simulink model "shunthybrid"  (Simulink 7.3)
settings: Solver=ode45  StartTime=0.0  StopTime=1.5  RelTol=1e-3
InitFcn:
  | Ts=50e-6;
StartFcn:
  | clear all
  | clc
  | Ts=2e-6
libraries: powerlib x35, powerlib_extras x7
settings Model: Creator=Anil  LastModifiedBy=SANTOSH

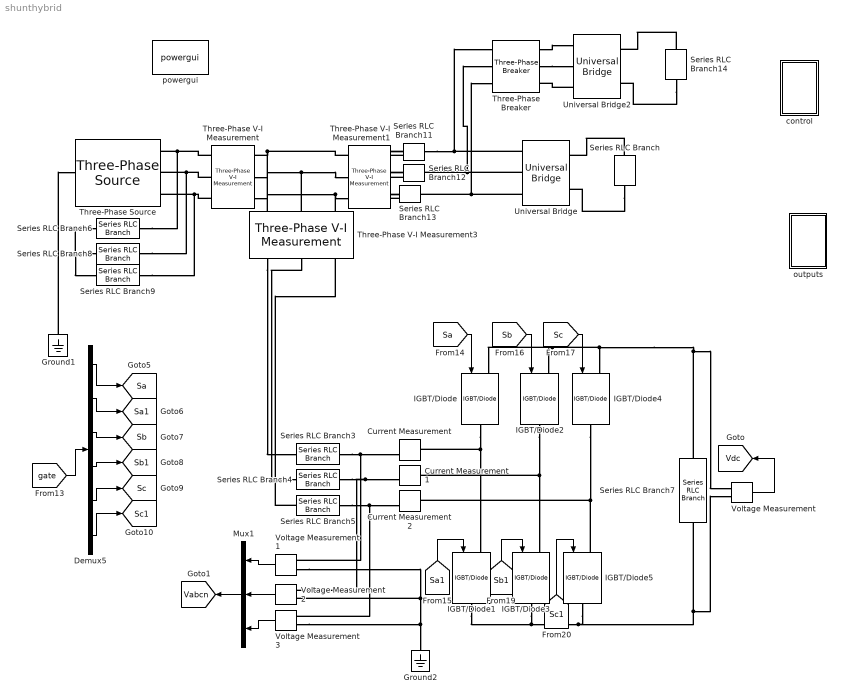
== system shunthybrid ==
  Current Measurement : powerlib/Measurements/Current Measurement  DialogController=POWERSYS.PowerSysDialog  SystemSampleTime=-1  PhasorSimulation=off  OutputType=Complex  PSBequivalent=0
  Current Measurement1 : powerlib/Measurements/Current Measurement  DialogController=POWERSYS.PowerSysDialog  SystemSampleTime=-1  PhasorSimulation=off  OutputType=Complex  PSBequivalent=0
  Current Measurement2 : powerlib/Measurements/Current Measurement  DialogController=POWERSYS.PowerSysDialog  SystemSampleTime=-1  PhasorSimulation=off  OutputType=Complex  PSBequivalent=0
  Demux5 : Demux  Outputs=6
  Ground1 : powerlib/Elements/Ground  DialogController=POWERSYS.PowerSysDialog  PhysicalDomain=powersysdomain  SubClassName=unknown  LeftPortType=p1  RightPortType=p1  LConnTagsString=a
  Ground2 : powerlib/Elements/Ground  DialogController=POWERSYS.PowerSysDialog  PhysicalDomain=powersysdomain  SubClassName=unknown  LeftPortType=p1  RightPortType=p1  LConnTagsString=a
  IGBT/Diode{,1..5} (6 alike) : powerlib/Power Electronics/IGBT//Diode  DialogController=POWERSYS.PowerSysDialog  SystemSampleTime=-1  Ron=1e-3  Rs=1e5  Cs=inf  Measurements=off
  Mux1 : Mux  Inputs=3
  Series RLC Branch : powerlib/Elements/Series RLC Branch  DialogController=POWERSYS.PowerSysDialog  PhysicalDomain=powersysdomain  SubClassName=unknown  LeftPortType=p1  RightPortType=p1  LConnTagsString=__new0  RConnTagsString=__new0  BranchType=R  Resistance=45  Inductance=1e-3  SetiL0=off  InitialCurrent=0  Capacitance=1e-6  Setx0=off  InitialVoltage=0  Measurements=None
  Series RLC Branch11 : powerlib/Elements/Series RLC Branch  DialogController=POWERSYS.PowerSysDialog  PhysicalDomain=powersysdomain  SubClassName=unknown  LeftPortType=p1  RightPortType=p1  LConnTagsString=__new0  RConnTagsString=__new0  BranchType=L  Resistance=75  Inductance=1.5e-3  SetiL0=off  InitialCurrent=0  Capacitance=1e-6  Setx0=off  InitialVoltage=0  Measurements=None
  Series RLC Branch12 : powerlib/Elements/Series RLC Branch  DialogController=POWERSYS.PowerSysDialog  PhysicalDomain=powersysdomain  SubClassName=unknown  LeftPortType=p1  RightPortType=p1  LConnTagsString=__new0  RConnTagsString=__new0  BranchType=L  Resistance=75  Inductance=1.5e-3  SetiL0=off  InitialCurrent=0  Capacitance=1e-6  Setx0=off  InitialVoltage=0  Measurements=None
  Series RLC Branch13 : powerlib/Elements/Series RLC Branch  DialogController=POWERSYS.PowerSysDialog  PhysicalDomain=powersysdomain  SubClassName=unknown  LeftPortType=p1  RightPortType=p1  LConnTagsString=__new0  RConnTagsString=__new0  BranchType=L  Resistance=75  Inductance=1.5e-3  SetiL0=off  InitialCurrent=0  Capacitance=1e-6  Setx0=off  InitialVoltage=0  Measurements=None
  Series RLC Branch14 : powerlib/Elements/Series RLC Branch  DialogController=POWERSYS.PowerSysDialog  PhysicalDomain=powersysdomain  SubClassName=unknown  LeftPortType=p1  RightPortType=p1  LConnTagsString=__new0  RConnTagsString=__new0  BranchType=R  Resistance=45  Inductance=1e-3  SetiL0=off  InitialCurrent=0  Capacitance=1e-6  Setx0=off  InitialVoltage=0  Measurements=None
  Series RLC Branch3 : powerlib/Elements/Series RLC Branch  DialogController=POWERSYS.PowerSysDialog  PhysicalDomain=powersysdomain  SubClassName=unknown  LeftPortType=p1  RightPortType=p1  LConnTagsString=__new0  RConnTagsString=__new0  BranchType=RL  Resistance=0.6  Inductance=5e-3  SetiL0=off  InitialCurrent=0  Capacitance=1e-6  Setx0=off  InitialVoltage=0  Measurements=None
  Series RLC Branch4 : powerlib/Elements/Series RLC Branch  DialogController=POWERSYS.PowerSysDialog  PhysicalDomain=powersysdomain  SubClassName=unknown  LeftPortType=p1  RightPortType=p1  LConnTagsString=__new0  RConnTagsString=__new0  BranchType=RL  Resistance=0.6  Inductance=5e-3  SetiL0=off  InitialCurrent=0  Capacitance=1e-6  Setx0=off  InitialVoltage=0  Measurements=None
  Series RLC Branch5 : powerlib/Elements/Series RLC Branch  DialogController=POWERSYS.PowerSysDialog  PhysicalDomain=powersysdomain  SubClassName=unknown  LeftPortType=p1  RightPortType=p1  LConnTagsString=__new0  RConnTagsString=__new0  BranchType=RL  Resistance=0.6  Inductance=5e-3  SetiL0=off  InitialCurrent=0  Capacitance=1e-6  Setx0=off  InitialVoltage=0  Measurements=None
  Series RLC Branch6 : powerlib/Elements/Series RLC Branch  DialogController=POWERSYS.PowerSysDialog  PhysicalDomain=powersysdomain  SubClassName=unknown  LeftPortType=p1  RightPortType=p1  LConnTagsString=__new0  RConnTagsString=__new0  BranchType=RC  Resistance=5  Inductance=5e-3  SetiL0=off  InitialCurrent=0  Capacitance=5e-6  Setx0=off  InitialVoltage=0  Measurements=None
  Series RLC Branch7 : powerlib/Elements/Series RLC Branch  DialogController=POWERSYS.PowerSysDialog  PhysicalDomain=powersysdomain  SubClassName=unknown  LeftPortType=p1  RightPortType=p1  LConnTagsString=__new0  RConnTagsString=__new0  BranchType=C  Resistance=0.6  Inductance=5e-3  SetiL0=off  InitialCurrent=0  Capacitance=2200e-6  Setx0=off  InitialVoltage=0  Measurements=None
  Series RLC Branch8 : powerlib/Elements/Series RLC Branch  DialogController=POWERSYS.PowerSysDialog  PhysicalDomain=powersysdomain  SubClassName=unknown  LeftPortType=p1  RightPortType=p1  LConnTagsString=__new0  RConnTagsString=__new0  BranchType=RC  Resistance=5  Inductance=5e-3  SetiL0=off  InitialCurrent=0  Capacitance=5e-6  Setx0=off  InitialVoltage=0  Measurements=None
  Series RLC Branch9 : powerlib/Elements/Series RLC Branch  DialogController=POWERSYS.PowerSysDialog  PhysicalDomain=powersysdomain  SubClassName=unknown  LeftPortType=p1  RightPortType=p1  LConnTagsString=__new0  RConnTagsString=__new0  BranchType=RC  Resistance=5  Inductance=5e-3  SetiL0=off  InitialCurrent=0  Capacitance=5e-6  Setx0=off  InitialVoltage=0  Measurements=None
  Three-Phase V-I Measurement : powerlib/Measurements/Three-Phase V-I Measurement  DialogController=POWERSYS.PowerSysDialog  SystemSampleTime=-1  VoltageMeasurement=phase-to-ground  SetLabelV=on  LabelV=Vsabc  Vpu=off  CurrentMeasurement=yes  SetLabelI=on  LabelI=Isabc  Ipu=off  Pbase=100e6  Vbase=500e3  OutputType=Complex  PhasorSimulation=off  PSBequivalent=0
  Three-Phase V-I Measurement1 : powerlib/Measurements/Three-Phase V-I Measurement  DialogController=POWERSYS.PowerSysDialog  SystemSampleTime=-1  VoltageMeasurement=phase-to-ground  SetLabelV=on  LabelV=VLabc  Vpu=off  CurrentMeasurement=yes  SetLabelI=on  LabelI=ILabc  Ipu=off  Pbase=100e6  Vbase=500e3  OutputType=Complex  PhasorSimulation=off  PSBequivalent=0
  Three-Phase V-I Measurement3 : powerlib/Measurements/Three-Phase V-I Measurement  DialogController=POWERSYS.PowerSysDialog  SystemSampleTime=-1  VoltageMeasurement=phase-to-ground  SetLabelV=on  LabelV=Vo  Vpu=off  CurrentMeasurement=yes  SetLabelI=on  LabelI=Iou  Ipu=off  Pbase=100e6  Vbase=500e3  OutputType=Complex  PhasorSimulation=off  PSBequivalent=0
  Three-Phase Breaker : powerlib/Elements/Three-Phase Breaker  DialogController=POWERSYS.PowerSysDialog  SystemSampleTime=-1  InitialState=open  SwitchA=on  SwitchB=on  SwitchC=on  SwitchTimes=[0.6]  External=off  BreakerResistance=0.001  SnubberResistance=1e6  SnubberCapacitance=inf  Measurements=None
  Three-Phase Source : powerlib/Electrical Sources/Three-Phase Source  DialogController=POWERSYS.PowerSysDialog  SystemSampleTime=-1  Voltage=55*sqrt(3)  PhaseAngle=0  Frequency=50  InternalConnection=Yn  SpecifyImpedance=on  Resistance=0.2  Inductance=1e-3  ShortCircuitLevel=100e3  BaseVoltage=55*sqrt(3)  XRratio=3
  Universal Bridge : powerlib/Power Electronics/Universal Bridge  DialogController=POWERSYS.PowerSysDialog  SystemSampleTime=-1  Arms=3  SnubberResistance=1e5  SnubberCapacitance=inf  Device=Diodes  Ron=1e-3  Lon=0  ForwardVoltages="[  0  0  ]"  ForwardVoltage=0  GTOparameters=[ 10e-6 , 20e-6 ]  IGBTparameters=[ 1e-6 , 2e-6 ]  Measurements=None  Measurements_2=None  converterType=Rectifier
  Universal Bridge2 : powerlib/Power Electronics/Universal Bridge  DialogController=POWERSYS.PowerSysDialog  SystemSampleTime=-1  Arms=3  SnubberResistance=1e5  SnubberCapacitance=inf  Device=Diodes  Ron=1e-3  Lon=0  ForwardVoltages="[  0  0  ]"  ForwardVoltage=0  GTOparameters=[ 10e-6 , 20e-6 ]  IGBTparameters=[ 1e-6 , 2e-6 ]  Measurements=None  Measurements_2=None  converterType=Rectifier
  Voltage Measurement{,1..3} (4 alike) : powerlib/Measurements/Voltage Measurement  DialogController=POWERSYS.PowerSysDialog  SystemSampleTime=-1  PhasorSimulation=off  OutputType=Complex  PSBequivalent=0
  control : Subsystem
  outputs : Subsystem
  powergui : powerlib/powergui  Priority=1  SystemSampleTime=-1  SimulationMode=Discrete  SampleTime=50e-6  frequency=60  SPID=off  DisableSnubberDevices=off  DisableRonSwitches=off  DisableVfSwitches=off  SwTol=0  Interpol=off  frequencyindice=50  echomessages=off  HookPort=off  DisplayEquations=off  FunctionMessages=off  EnableUseOfTLC=off  x0status=blocks  RestoreLinks=warning  Frange=[0:2:500]  Ylog=off  Xlog=on  ShowGrid=off  save=off  variable=ZData  structure=ScopeData  ZoomFFT=on  StartTime=0.1  cycles=10  DisplayStyle=1  fundamental=50  FreqAxis=off  MaxFrequency=1000  frequencyindicesteady=1  RmsSteady=1  display=off  Ts=0  methode=off
  tag scope: Sa1=global, Sa=global, Sb1=global, Sb=global, Sc1=global, Sc=global, Vabcn=global, Vdc=global
  wires:
  Voltage Measurement/1 -> [Vdc]
  [gate] -> Demux5/1
  Demux5/1 -> [Sa]
  Demux5/2 -> [Sa1]
  Demux5/3 -> [Sb]
  Demux5/4 -> [Sb1]
  Demux5/5 -> [Sc]
  Demux5/6 -> [Sc1]
  [Sa] -> IGBT/Diode/1
  [Sa1] -> IGBT/Diode1/1
  [Sb] -> IGBT/Diode2/1
  [Sc] -> IGBT/Diode4/1
  [Sb1] -> IGBT/Diode3/1
  [Sc1] -> IGBT/Diode5/1
  Voltage Measurement1/1 -> Mux1/1
  Voltage Measurement2/1 -> Mux1/2
  Voltage Measurement3/1 -> Mux1/3
  Mux1/1 -> [Vabcn]
  connections:
  Ground1/LConn1 -- Three-Phase Source/LConn1
  Three-Phase V-I Measurement/LConn1 -- Three-Phase Source/RConn1 -- Series RLC Branch6/RConn1
  Three-Phase V-I Measurement/LConn2 -- Three-Phase Source/RConn2 -- Series RLC Branch8/RConn1
  Three-Phase V-I Measurement/LConn3 -- Three-Phase Source/RConn3 -- Series RLC Branch9/RConn1
  Three-Phase V-I Measurement3/RConn1 -- Three-Phase V-I Measurement1/LConn1 -- Three-Phase V-I Measurement/RConn1
  Three-Phase V-I Measurement3/RConn2 -- Three-Phase V-I Measurement/RConn2 -- Three-Phase V-I Measurement1/LConn2
  Three-Phase V-I Measurement3/RConn3 -- Three-Phase V-I Measurement/RConn3 -- Three-Phase V-I Measurement1/LConn3
  Universal Bridge/LConn1 -- Series RLC Branch11/LConn1 -- Three-Phase Breaker/LConn1
  Series RLC Branch/LConn1 -- Universal Bridge/RConn1
  Series RLC Branch/RConn1 -- Universal Bridge/RConn2
  Current Measurement/LConn1 -- IGBT/Diode/RConn1 -- IGBT/Diode1/LConn1
  Current Measurement1/LConn1 -- IGBT/Diode2/RConn1 -- IGBT/Diode3/LConn1
  IGBT/Diode5/LConn1 -- IGBT/Diode4/RConn1 -- Current Measurement2/LConn1
  IGBT/Diode/LConn1 -- IGBT/Diode2/LConn1 -- IGBT/Diode4/LConn1 -- Series RLC Branch7/LConn1 -- Voltage Measurement/LConn1
  IGBT/Diode1/RConn1 -- IGBT/Diode3/RConn1 -- IGBT/Diode5/RConn1 -- Series RLC Branch7/RConn1 -- Voltage Measurement/LConn2
  Series RLC Branch3/RConn1 -- Current Measurement/RConn1 -- Voltage Measurement1/LConn1
  Series RLC Branch4/RConn1 -- Current Measurement1/RConn1 -- Voltage Measurement2/LConn1
  Series RLC Branch5/RConn1 -- Current Measurement2/RConn1 -- Voltage Measurement3/LConn1
  Three-Phase V-I Measurement3/LConn2 -- Series RLC Branch4/LConn1
  Series RLC Branch5/LConn1 -- Three-Phase V-I Measurement3/LConn3
  Series RLC Branch8/LConn1 -- Series RLC Branch9/LConn1 -- Series RLC Branch6/LConn1
  Three-Phase V-I Measurement3/LConn1 -- Series RLC Branch3/LConn1
  Voltage Measurement3/LConn2 -- Voltage Measurement1/LConn2 -- Voltage Measurement2/LConn2 -- Ground2/LConn1
  Series RLC Branch11/RConn1 -- Three-Phase V-I Measurement1/RConn1
  Series RLC Branch12/RConn1 -- Three-Phase V-I Measurement1/RConn2
  Universal Bridge/LConn2 -- Series RLC Branch12/LConn1 -- Three-Phase Breaker/LConn2
  Series RLC Branch13/RConn1 -- Three-Phase V-I Measurement1/RConn3
  Universal Bridge/LConn3 -- Series RLC Branch13/LConn1 -- Three-Phase Breaker/LConn3
  Series RLC Branch14/LConn1 -- Universal Bridge2/RConn1
  Series RLC Branch14/RConn1 -- Universal Bridge2/RConn2
  Universal Bridge2/LConn3 -- Three-Phase Breaker/RConn3
  Three-Phase Breaker/RConn2 -- Universal Bridge2/LConn2
  Three-Phase Breaker/RConn1 -- Universal Bridge2/LConn1

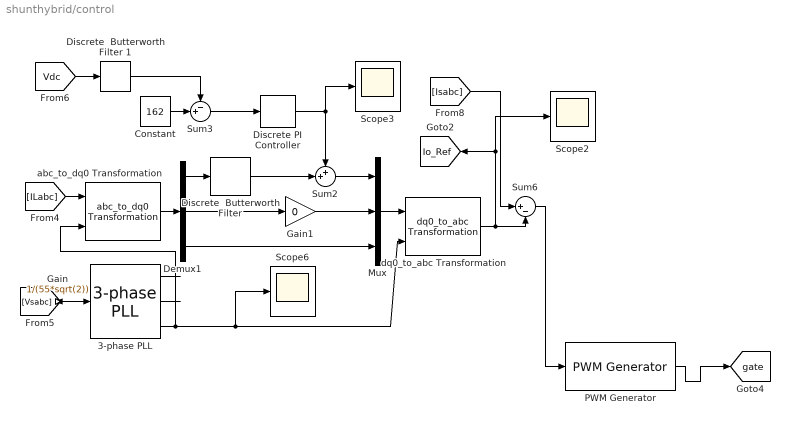
== system shunthybrid/control ==
  3-phase PLL : powerlib_extras/Control  Blocks/3-phase PLL  DialogController=POWERSYS.PowerSysDialog  SystemSampleTime=-1  Par_Init=[0 50]  ParK=[ 180 3200 1 ]  AGC=off
  Constant : Constant  Value=162  OutDataType=fixdt(1, 16)  OutScaling=2^0
  Demux1 : Demux  Outputs=3
  Discrete PI Controller : powerlib_extras/Discrete  Control Blocks/Discrete PI Controller  DialogController=POWERSYS.PowerSysDialog  SystemSampleTime=-1  Kp=0.1  Ki=0.32  Par_Limits=[1e6 -1e6]  Init=0  Ts=Ts
  "Discrete  Butterworth Filter " : powerlib_extras/Discrete  Control Blocks/Discrete  Butterworth Filter   DialogController=POWERSYS.PowerSysDialog  SystemSampleTime=-1  FilterType=Lowpass  N=2  Fo=20  Bo=5  Ts=Ts  Initialize=off  Vac_Init=[1.2 60 60]  Vdc_Init=-0.6  PlotResponse=off  param1=[1 500 0.1]
  Discrete  Butterworth Filter 1 : powerlib_extras/Discrete  Control Blocks/Discrete  Butterworth Filter   DialogController=POWERSYS.PowerSysDialog  SystemSampleTime=-1  FilterType=Lowpass  N=2  Fo=16  Bo=5  Ts=Ts  Initialize=off  Vac_Init=[1.2 60 60]  Vdc_Init=-0.6  PlotResponse=off  param1=[1 500 0.1]
  Gain : Gain  Gain=1/(55*sqrt(2))  ParameterDataType=fixdt(1, 16)  ParameterScaling=2^0  OutDataType=fixdt(1, 16)  OutScaling=2^0
  Gain1 : Gain  Gain=0  ParameterDataType=fixdt(1, 16)  ParameterScaling=2^0  OutDataType=fixdt(1, 16)  OutScaling=2^0
  Mux : Mux  Inputs=3
  PWM Generator : powerlib_extras/Control  Blocks/PWM Generator  DialogController=POWERSYS.PowerSysDialog  SystemSampleTime=-1  GeneratorMode="3-arm  bridge (6 pulses)"  Fc=12000  Internal=off  mIndex=0.4  Freq=60  Phase=0
  Scope2 : Scope
      settings: YMin=-2.25  YMax=2.25  SaveName=ScopeData2
  Scope3 : Scope
      settings: YMin=13.7  YMax=15.2  SaveName=ScopeData3
  Scope6 : Scope
      settings: YMin=-1  YMax=1  SaveName=ScopeData6
  Sum2 : Sum  Inputs=++|  OutDataType=fixdt(1, 16)  OutScaling=2^0
  Sum3 : Sum  Inputs=-+|  OutDataType=fixdt(1, 16)  OutScaling=2^0
  Sum6 : Sum  Inputs=|+-  OutDataType=fixdt(1, 16)  OutScaling=2^0
  abc_to_dq0 Transformation : powerlib_extras/Measurements/abc_to_dq0 Transformation  DialogController=POWERSYS.PowerSysDialog  SystemSampleTime=-1
  dq0_to_abc Transformation : powerlib_extras/Measurements/dq0_to_abc Transformation  DialogController=POWERSYS.PowerSysDialog  SystemSampleTime=-1
  tag scope: Io_Ref=global, gate=global
  wires:
  [Vsabc] -> Gain/1
  Constant/1 -> Sum3/2
  Gain/1 -> 3-phase PLL/1
  [ILabc] -> abc_to_dq0 Transformation/1
  3-phase PLL/3 -> abc_to_dq0 Transformation/2, dq0_to_abc Transformation/2, Scope6/1
  abc_to_dq0 Transformation/1 -> Demux1/1
  Demux1/1 -> "Discrete  Butterworth Filter "/1
  "Discrete  Butterworth Filter "/1 -> Sum2/2
  [Vdc] -> Discrete  Butterworth Filter 1/1
  Sum3/1 -> Discrete PI Controller/1
  Discrete PI Controller/1 -> Sum2/1, Scope3/1
  Demux1/2 -> Gain1/1
  Sum2/1 -> Mux/1
  Gain1/1 -> Mux/2
  Demux1/3 -> Mux/3
  Mux/1 -> dq0_to_abc Transformation/1
  dq0_to_abc Transformation/1 -> Sum6/2, [Io_Ref], Scope2/1
  Discrete  Butterworth Filter 1/1 -> Sum3/1
  Sum6/1 -> PWM Generator/1
  [Isabc] -> Sum6/1
  PWM Generator/1 -> [gate]
  3-phase PLL/1 -> ?
  3-phase PLL/2 -> ?

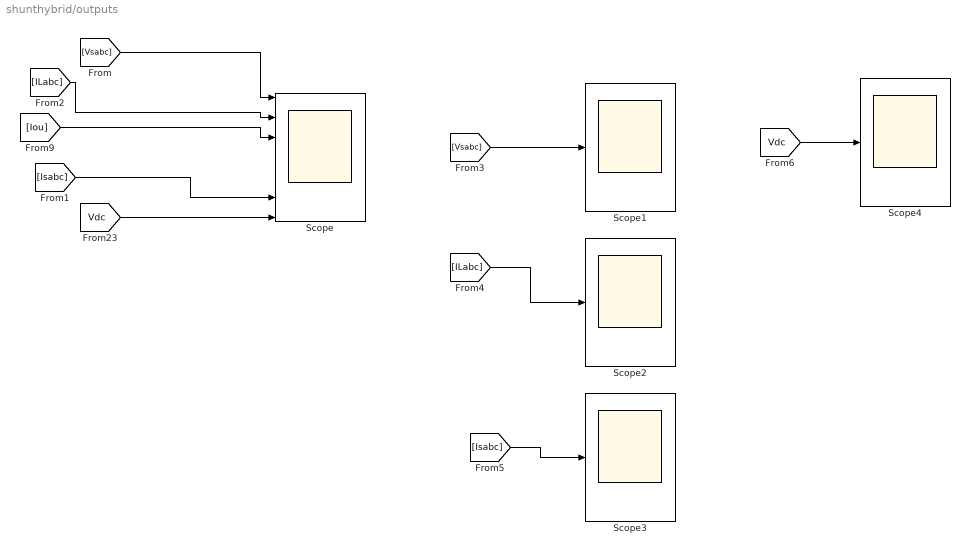
== system shunthybrid/outputs ==
  Scope : Scope  NumInputPorts=7
      settings: YMin=-100~-7.5~-5~-1~-1~-10~152.5  YMax=100~7.5~5~1~1~10~170  SaveName=ScopeData2
  Scope{1..4} (4 alike) : Scope
      Scope1 settings: YMin=-100  YMax=100
      Scope2 settings: YMin=-100  YMax=100
      Scope3 settings: YMin=-100  YMax=100  SaveName=ScopeData4
      Scope4 settings: YMin=162.25  YMax=165.5  SaveName=ScopeData5
  wires:
  [Vsabc] -> Scope/1
  [ILabc] -> Scope/2
  [Iou] -> Scope/3
  [Vdc] -> Scope/7
  [Isabc] -> Scope/6
  ? -> Scope/4
  ? -> Scope/5
  [Vsabc] -> Scope1/1
  [ILabc] -> Scope2/1
  [Isabc] -> Scope3/1
  [Vdc] -> Scope4/1
